simulink model "SS_OBSERVER"  (R2019b)
settings: Solver=VariableStepAuto  StartTime=0.0  StopTime=0.005  RelTol=1e-3  EnableMultiTasking=on
undefined symbols (not defined in the file): K2, L2, sigbuilder_block, sysog
settings Model: Creator=zap  LastModifiedBy=bhisma
settings DataIOCC: LimitDataPoints=on  ReturnWorkspaceOutputs=off
settings OptimizationCC: LifeSpan=inf
settings DebuggingCC: AllowSymbolicDim=off  SFUnexpectedBacktrackingDiag=warning  SFNoUnconditionalDefaultTransitionDiag=warning  SFExecutionAtInitializationDiag=none  ArithmeticOperatorsInVariantConditions=warning
settings ModelReferenceCC: PropagateSignalLabelsOutOfModel=off
settings SFSimCC: SimUseLocalCustomCode=off  CustomCodeUndefinedFunction=UseInterfaceOnly
settings RTWCC: RTWUseLocalCustomCode=off
settings CodeAppCC: StateflowObjectComments=on
settings GRTTargetCC: TargetLangStandard=C89/C90 (ANSI)
settings ConfigComp: CovMetricSettings=dw  CovHtmlReporting=on  CovSaveCumulativeToWorkspaceVar=on  CovSaveSingleToWorkspaceVar=on  CovExternalEMLEnable=off

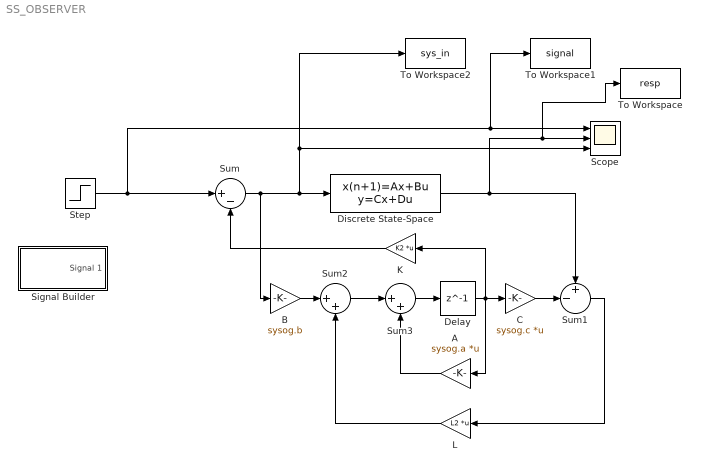
== system SS_OBSERVER ==
  A : Gain  Gain=sysog.a  Multiplication=Matrix(K*u)
  B : Gain  Gain=sysog.b
  C : Gain  Gain=sysog.c  Multiplication=Matrix(K*u)
  Delay : Delay  DelayLength=1  InitialCondition=0
  Discrete State-Space : DiscreteStateSpace  A=sysog.a  B=sysog.b  C=sysog.c  D=sysog.d  SampleTime=10^-4
  K : Gain  Gain=K2  Multiplication=Matrix(K*u)
  L : Gain  Gain=L2  Multiplication=Matrix(K*u)
  Scope : Scope  NumInputPorts=3
  Signal Builder : Subsystem  Tag=STV Subsys  LoadFcn=sigbuilder_block('load');  StartFcn=sigbuilder_block('start');  StopFcn=sigbuilder_block('stop');  ClipboardFcn=sigbuilder_block('clipboard');  mask(Sigbuilder block){tuvar=[0:10]}
      mask help: Simulink:masks:SigbuilderBlock_MD
      mask init:
      | if ~strcmp(get_param(bdroot(gcbh),'SimulationStatus'),'stopped') tuvar = sigbuilder_block('maskInit'); end
      settings: CopyFcn=sigbuilder_block('copy');  DeleteFcn=sigbuilder_block('delete');  ModelCloseFcn=sigbuilder_block('modelClose');  PreSaveFcn=sigbuilder_block('preSave');  PauseFcn=sigbuilder_block('pause');  ContinueFcn=sigbuilder_block('continue');  NameChangeFcn=sigbuilder_block('namechange');  OpenFcn=sigbuilder_block('open',[437.25 199.5 550.5 399.75 ]);  CloseFcn=sigbuilder_block('close');
      mask Display: plot(0, 0, 100, 100,[2, 2, 32, 32, 2], [68, 8, 8, 68, 68],[32, 2], [38, 38], [32, 19, 2],[53, 60, 44], [32, 17, 17, 2],[16, 16, 31, 31]);txt = getActiveGroup(gcbh);text(2, 100, txt,'verticalAlignment', 'top');
  Step : Step  Time=0  After=1/57  SampleTime=10^-4
  Sum : Sum  Inputs=|+-
  Sum1 : Sum  Inputs=+-|
  Sum2 : Sum  Inputs=|++
  Sum3 : Sum  Inputs=|++
  To Workspace : ToWorkspace  VariableName=resp  SaveFormat=Timeseries  SampleTime=-1
  To Workspace1 : ToWorkspace  VariableName=signal  SaveFormat=Timeseries  SampleTime=-1
  To Workspace2 : ToWorkspace  VariableName=sys_in  SaveFormat=Timeseries  SampleTime=-1
  wires:
  Discrete State-Space/1 -> Sum1/1, To Workspace/1, Scope/2
  Sum/1 -> B/1, To Workspace2/1, Scope/3, Discrete State-Space/1
  B/1 -> Sum2/1
  Sum2/1 -> Sum3/1
  Sum3/1 -> Delay/1
  A/1 -> Sum3/2
  Delay/1 -> K/1, C/1, A/1
  C/1 -> Sum1/2
  Sum1/1 -> L/1
  L/1 -> Sum2/2
  K/1 -> Sum/2
  Step/1 -> To Workspace1/1, Scope/1, Sum/1

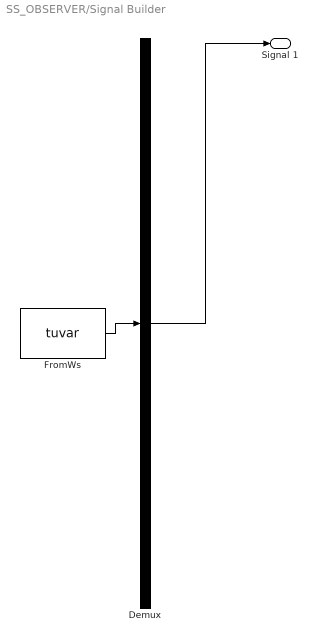
== system SS_OBSERVER/Signal Builder ==
  Demux : Demux  Tag=STV Demux  Outputs=1
  FromWs : FromWorkspace  Tag=STV FromWs  VariableName=tuvar  SampleTime=10^(-4)  OutputAfterFinalValue=Holding final value
      SigBuilderData=|
      | common.afterFinalStr = 'Hold final value'
      | common.sampleTime = '10^(-4)'
      | dataSet.timeRange = [0 0.15]
      | dataSet.name = 'Group 1'
      | sbobj.Groups.Name = 'Group 1'
      | sbobj.Groups.Signals.Name = 'Signal 1'
      | sbobj.Groups.Signals.XData = [0 0.025 0.05 0.075 0.1 0.15]
      | sbobj.Groups.Signals.YData = [0 0.0175438596491 0 0.0175438596491 0 0]
      | sbobj.Groups.TimeRange = [0 0.15]
  Signal 1 : Outport  Tag=STV Outport
  wires:
  Demux/1 -> Signal 1/1
  FromWs/1 -> Demux/1
